simulink library "simetranss"  (R2024b)
settings: Solver=VariableStepAuto  StartTime=0.0  StopTime=10.0  RelTol=1e-3
PostLoadFcn:
  | Ts=1e-6
InitFcn:
  | Ts=1e-6
undefined symbols (not defined in the file): C, C_601, C_603, C_606, CC, Csnu, Csnubber, DiscIntNeverNeededParam, DPL, DPL1ph, FluxTable, ft2km, gcbh, h, Half, Imap2, L, L_601, L_603, L_606, Lbase, LpejoSw, Newton, R_601, R_603, R_606, Raphson, ResistanceM, Roff, Ron, RotorAngles, Rsnu, Rsnubber, Rt4, SampleTime, simetran, sps, sps_rtmsupport, StatorCurrents, T_2wind_ratio, T_Lpu, T_Lpu_pri, T_Rpu, T_Rpu_pri, T_Vpri, T_Vpri_15comp, T_Vsec, Ti, Ts_Power, Z, Zbase, Zm
libraries: fl_lib x248, ee_lib x146, nesl_utility x122, $bdroot x29, simulink x15, eeGeneralControl x2, spsStairGeneratorLib x2, artemis x1
(part 6 of 12)

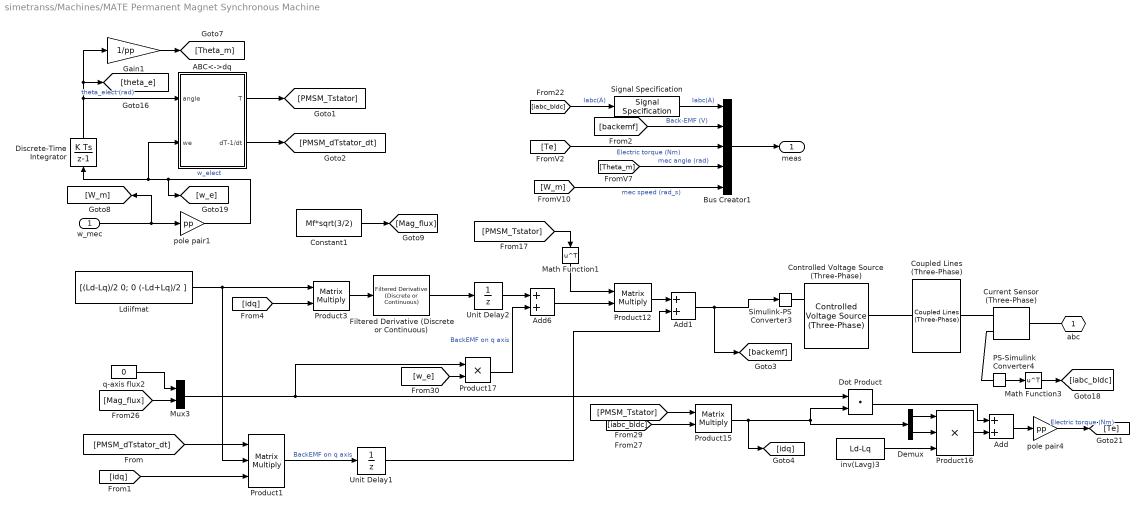
== system simetranss/Machines/MATE Permanent Magnet Synchronous Machine ==
  "   w_mec" : Inport
  ABC<->dq : Subsystem
  Add : Sum
  Add1 : Sum  Inputs=2
  Add6 : Sum  Inputs=2
  Bus Creator1 : BusCreator  Inputs=5
  Constant1 : Constant  Value=Mf*sqrt(3/2)
  Controlled Voltage Source (Three-Phase) : ee_lib/Sources/Controlled Voltage Source (Three-Phase)  input_option=ee.enum.inputType.instantaneous  FRated=60 Hz
      settings: InternalSimscapePortConfiguration="{\"Bottom\":[],\"Left\":[{\"id\":\"S\",\"label\":\"S\",\"type\":\"input\"},{\"id\":\"n\",\"label\":\"n\",\"type\":\"foundation.electrical.electrical\"}],\"Right\":[{\"id\":\"N\",\"label\":\"~\",\"type\":\"foundation.electrical.three_phase\"}],\"Top\":[]}"
  Coupled Lines (Three-Phase) : ee_lib/Passive/Lines/Coupled Lines (Three-Phase)  prm=1  La=1e-3 H  Lb=1e-3 H  Lc=1e-3 H  L=Ld+Lq H  Lmab=3e-4 H  Lmac=3e-4 H  Lmbc=3e-4 H  Lm=(Ld+Lq)/2 H  Ra=0.001 Ohm  Rb=0.001 Ohm  Rc=0.001 Ohm  R=Rs Ohm  Rm=0 Ohm  Ga=1e-9 1/Ohm  Gb=1e-9 1/Ohm  Gc=1e-9 1/Ohm  G=1e-9 1/Ohm  I_L_specify=off  I_L_priority=High  I_L=[0, 0, 0] A  I_L_nominal_specify=off  I_L_nominal_value=1  I_L_nominal_unit=A  i_La_specify=off  i_La_priority=High  i_La=0 A  i_La_nominal_specify=off  i_La_nominal_value=1  i_La_nominal_unit=A  i_Lb_specify=off  i_Lb_priority=High  i_Lb=0 A  i_Lb_nominal_specify=off  i_Lb_nominal_value=1  i_Lb_nominal_unit=A  i_Lc_specify=off  i_Lc_priority=High  i_Lc=0 A  i_Lc_nominal_specify=off  i_Lc_nominal_value=1  i_Lc_nominal_unit=A
      settings: InternalSimscapePortConfiguration="{\"Bottom\":[],\"Left\":[{\"id\":\"N1\",\"label\":\"~1\",\"type\":\"foundation.electrical.three_phase\"}],\"Right\":[{\"id\":\"N2\",\"label\":\"~2\",\"type\":\"foundation.electrical.three_phase\"}],\"Top\":[]}"
  Current Sensor (Three-Phase) : ee_lib/Sensors & Transducers/Current Sensor (Three-Phase)
  Demux : Demux  Outputs=2
  Discrete-Time Integrator : DiscreteIntegrator  InitialCondition=pp*AngInit/180*pi  SampleTime=Ts  ICPrevOutput=DiscIntNeverNeededParam  ICPrevScaledInput=DiscIntNeverNeededParam
  Dot Product : DotProduct  OutDataTypeStr=Inherit: Inherit via internal rule
  Filtered Derivative (Discrete or Continuous) : eeGeneralControl/Filtered Derivative (Discrete or Continuous)  K=1  T=sal_der  B=inf  A=-inf  minRatio=10  init_option=Inherited from block input  x0=0  Ts=Ts
  Gain1 : Gain  Gain=1/pp
  Ldiifmat : Constant  Value=[(Ld-Lq)/2 0; 0 (-Ld+Lq)/2 ]
  Math Function1 : Math  Operator=transpose  SignedPower=on
  Math Function3 : Math  Operator=transpose  SignedPower=on
  Mux3 : Mux  Inputs=2
  PS-Simulink Converter4 : nesl_utility/PS-Simulink Converter  PhysicalDomain=network_engine_domain  SubClassName=ps_output  LeftPortType=input  RightPortType=output  PseudoPeriodic=off  Frequencies=[]  VectorFormat=inherit  Unit=inherit  AffineConversion=off
  Product1 : Product  Inputs=3  Multiplication=Matrix(*)  SaturateOnIntegerOverflow=on  OutDataTypeStr=Inherit: Same as first input
  Product12 : Product  Multiplication=Matrix(*)  SaturateOnIntegerOverflow=on  OutDataTypeStr=Inherit: Same as first input
  Product15 : Product  Multiplication=Matrix(*)  SaturateOnIntegerOverflow=on  OutDataTypeStr=Inherit: Same as first input
  Product16 : Product  Inputs=3  SaturateOnIntegerOverflow=on  OutDataTypeStr=Inherit: Same as first input
  Product17 : Product  RndMeth=Zero
  Product3 : Product  Multiplication=Matrix(*)  SaturateOnIntegerOverflow=on  OutDataTypeStr=Inherit: Same as first input
  Signal Specification : SignalSpecification  Dimensions=3
  Simulink-PS Converter3 : nesl_utility/Simulink-PS Converter  PhysicalDomain=network_engine_domain  SubClassName=ps_input  LeftPortType=input  RightPortType=output  PseudoPeriodic=off  Frequencies=[]  NoiseDistribution=none  NoiseParameters=[]  Unit=1  AffineConversion=off  FilteringAndDerivatives=provide  SimscapeFilterOrder=1  InputFilterTimeConstant=0.001  UdotUserProvided=0
  Unit Delay1 : UnitDelay  SampleTime=Ts  HasFrameUpgradeWarning=on
  Unit Delay2 : UnitDelay  SampleTime=Ts  HasFrameUpgradeWarning=on
  inv(Lavg)3 : Constant  Value=Ld-Lq
  pole pair1 : Gain  Gain=pp
  pole pair4 : Gain  Gain=pp
  q-axis flux2 : Constant  Value=0
  "   abc" : PMIOPort  Side=Left
  meas : Outport  VectorParamsAs1DForOutWhenUnconnected=off
  wires:
  Unit Delay1/1 -> Add1/2
  [idq] -> Product3/2
  Product1/1 -> Unit Delay1/1  "BackEMF on q axis"
  Add1/1 -> Simulink-PS Converter3/1, [backemf]
  Product12/1 -> Add1/1
  [idq] -> Product1/3
  Ldiifmat/1 -> Product3/1, Product1/2
  [PMSM_dTstator_dt] -> Product1/1
  Add6/1 -> Product12/2
  Math Function1/1 -> Product12/1
  [PMSM_Tstator] -> Product15/1
  [iabc_bldc] -> Product15/2
  Math Function3/1 -> [iabc_bldc]
  [PMSM_Tstator] -> Math Function1/1
  ABC<->dq/2(dT-1/dt) -> [PMSM_dTstator_dt]
  Product17/1 -> Add6/2  "BackEMF on q axis"
  Unit Delay2/1 -> Add6/1
  Mux3/1 -> Product17/1, Dot Product/1
  [w_e] -> Product17/2
  Dot Product/1 -> Add/1
  Add/1 -> pole pair4/1
  Product16/1 -> Add/2
  pole pair4/1 -> [Te]  "Electric torque (Nm)"
  Demux/2 -> Product16/2
  Demux/1 -> Product16/1
  inv(Lavg)3/1 -> Product16/3
  Product15/1 -> Demux/1, Dot Product/2, [idq]
  Filtered Derivative (Discrete or Continuous)/1 -> Unit Delay2/1
  q-axis flux2/1 -> Mux3/1
  [Mag_flux] -> Mux3/2
  Product3/1 -> Filtered Derivative (Discrete or Continuous)/1
  [Te] -> Bus Creator1/3  "Electric torque (Nm)"
  [Theta_m] -> Bus Creator1/4  "mec angle (rad)"
  PS-Simulink Converter4/1 -> Math Function3/1
  [backemf] -> Bus Creator1/2  "Back-EMF (V)"
  Bus Creator1/1 -> meas/1
  Signal Specification/1 -> Bus Creator1/1  "Iabc(A)"
  [W_m] -> Bus Creator1/5  "mec speed (rad_s)"
  [iabc_bldc] -> Signal Specification/1  "Iabc(A)"
  Gain1/1 -> [Theta_m]
  Discrete-Time Integrator/1 -> ABC<->dq/1(angle), [theta_e], Gain1/1  "theta_elect (rad)"
  pole pair1/1 -> Discrete-Time Integrator/1, ABC<->dq/2(we), [w_e]  "w_elect"
  "   w_mec"/1 -> [W_m], pole pair1/1
  ABC<->dq/1(T) -> [PMSM_Tstator]
  Constant1/1 -> [Mag_flux]
  connections:
  PS-Simulink Converter4/LConn1 -- Current Sensor (Three-Phase)/RConn1
  Controlled Voltage Source (Three-Phase)/RConn1 -- Coupled Lines (Three-Phase)/RConn1
  Coupled Lines (Three-Phase)/LConn1 -- Current Sensor (Three-Phase)/RConn2
  Simulink-PS Converter3/RConn1 -- Controlled Voltage Source (Three-Phase)/LConn1
  Current Sensor (Three-Phase)/LConn1 -- "   abc"/RConn1

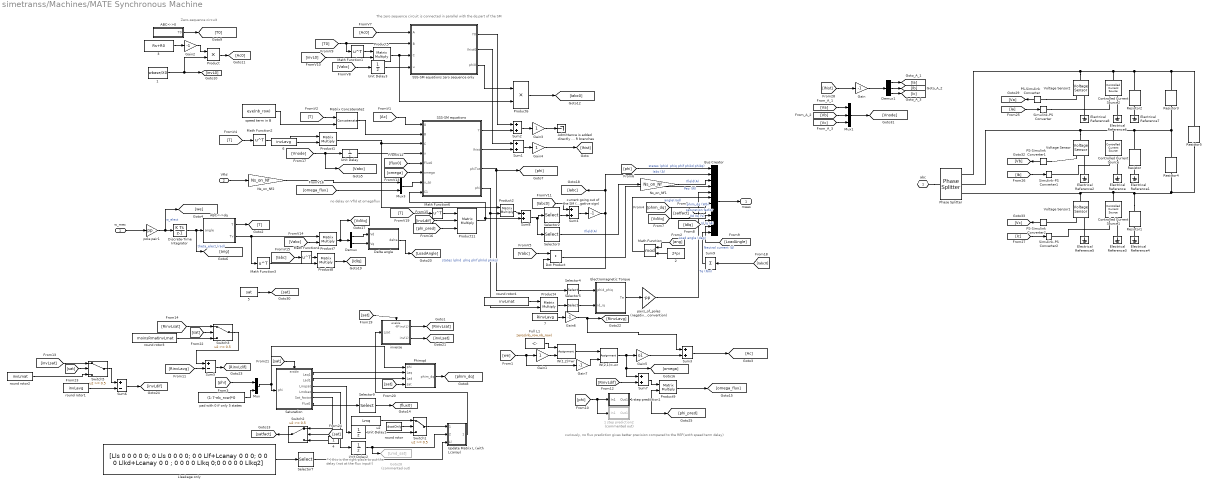
== system simetranss/Machines/MATE Synchronous Machine ==
  note: no delay on Vfld et omegaflux
  note: curiously, no flux prediction gives better precision compared to the REF(woth speed term delay)
  note: The zero sequence circuit is connected in parallel with the dq part of the SM
  note: Zero-sequence circuit
  note: ^
      | |
      | this is the right place to put the delay
      | (not at the flux input!)
  "   w_mec" : Inport
  "   Vfld" : Inport  Port=2
  1 : Constant  Value=wbase/X0
  1 step prediction1 : Subsystem
  1 step prediction2 : Subsystem  Commented=on
  2 : Constant  Value=2*pi
  3 : Constant  Value=Rs+R0
  4 : Constant
  5 : Constant  Value=sat
  6 : Constant  Value=invLavg
  7 : Constant  Value=RinvLavg
  ABC<->0 : Subsystem
  ABC<->dq : Subsystem
  Admittance is added directly with R branches : Terminator
  Bus Creator : BusCreator  Inputs=12
  Controlled Current Source : fl_lib/Electrical/Electrical Sources/Controlled Current Source
  Controlled Current Source1 : fl_lib/Electrical/Electrical Sources/Controlled Current Source
  Controlled Current Source2 : fl_lib/Electrical/Electrical Sources/Controlled Current Source
  Delta angle : Subsystem
  Demux : Demux  Outputs=2
  Demux1 : Demux  Outputs=3
      settings: DisplayOption=none
  Discrete-Time Integrator : DiscreteIntegrator  InitialCondition=theta_0  SampleTime=Ts  ICPrevOutput=DiscIntNeverNeededParam  ICPrevScaledInput=DiscIntNeverNeededParam
  Dot Product : DotProduct  OutDataTypeStr=Inherit: Inherit via internal rule
  Electrical Reference{,1..8} (9 alike) : fl_lib/Electrical/Electrical Elements/Electrical Reference
  Electromagnetic Torque : Subsystem
  Full L1 : Constant  Value=zeros(nb_row,nb_row)
  Gain : Gain  Gain=-1
  Gain1 : Gain  SaturateOnIntegerOverflow=on  OutDataTypeStr=Inherit: Same as input  ParamDataTypeStr=Inherit: Same as input
  Gain2 : Gain  Gain=-1
  Gain3 : Gain
  Gain4 : Gain
  Gain5 : Gain  Gain=o1
  Gain6 : Gain  Gain=-1
  Gain7 : Gain  Gain=-1  SaturateOnIntegerOverflow=on  OutDataTypeStr=Inherit: Same as input  ParamDataTypeStr=Inherit: Same as input
  Goto28 : Goto  Commented=on  GotoTag=Lmd_sat
  Lleakage only : Constant  Value="[Lls 0 0 0 0 0; 0 Lls 0 0  0 0; 0 0 Llf+Lcanay 0 0 0; 0 0 0 Llkd+Lcanay 0 0 ; 0 0 0 0 Llkq 0;0 0 0 0 0 Llkq2]"
  Math Function : Math  Operator=mod  SignedPower=on
  Math Function{1..4,6} (5 alike) : Math  Operator=transpose  SignedPower=on
  Matrix Concatenate2 : Concatenate  Mode=Multidimensional array  ConcatenateDimension=2
  Mux : Mux  Inputs=2
  Mux1 : Mux  Inputs=3
  Mux3 : Mux  Inputs=2
  Ns_on_Nf1 : Gain  Gain=Ns_on_Nf
  Ns_on_Nf2 : Gain  Gain=Ns_on_Nf
  PS-Simulink Converter : nesl_utility/PS-Simulink Converter  PhysicalDomain=network_engine_domain  SubClassName=ps_output  LeftPortType=input  RightPortType=output  PseudoPeriodic=off  Frequencies=[]  VectorFormat=inherit  Unit=inherit  AffineConversion=off
  PS-Simulink Converter1 : nesl_utility/PS-Simulink Converter  PhysicalDomain=network_engine_domain  SubClassName=ps_output  LeftPortType=input  RightPortType=output  PseudoPeriodic=off  Frequencies=[]  VectorFormat=inherit  Unit=inherit  AffineConversion=off
  PS-Simulink Converter2 : nesl_utility/PS-Simulink Converter  PhysicalDomain=network_engine_domain  SubClassName=ps_output  LeftPortType=input  RightPortType=output  PseudoPeriodic=off  Frequencies=[]  VectorFormat=inherit  Unit=inherit  AffineConversion=off
  Phase Splitter : ee_lib/Connectors & References/Phase Splitter
  Phimqd : Subsystem
  Product : Product  RndMeth=Zero
  Product{1..2,4..5,7..9} (7 alike) : Product  Multiplication=Matrix(*)  SaturateOnIntegerOverflow=on  OutDataTypeStr=Inherit: Same as first input
  Product11 : Product  Inputs=3  Multiplication=Matrix(*)  SaturateOnIntegerOverflow=on  OutDataTypeStr=Inherit: Same as first input
  Product6 : Product  SaturateOnIntegerOverflow=on  OutDataTypeStr=Inherit: Same as first input
  Resistor : fl_lib/Electrical/Electrical Elements/Resistor  R=ResistanceM(2,2) Ohm  i_specify=off  i_priority=None  i=0 A  i_nominal_specify=off  i_nominal_value=1  i_nominal_unit=A  v_specify=off  v_priority=None  v=0 V  v_nominal_specify=off  v_nominal_value=1  v_nominal_unit=V
  Resistor1 : fl_lib/Electrical/Electrical Elements/Resistor  R=ResistanceM(3,3) Ohm  i_specify=off  i_priority=None  i=0 A  i_nominal_specify=off  i_nominal_value=1  i_nominal_unit=A  v_specify=off  v_priority=None  v=0 V  v_nominal_specify=off  v_nominal_value=1  v_nominal_unit=V
  Resistor2 : fl_lib/Electrical/Electrical Elements/Resistor  R=ResistanceM(1,1) Ohm  i_specify=off  i_priority=None  i=0 A  i_nominal_specify=off  i_nominal_value=1  i_nominal_unit=A  v_specify=off  v_priority=None  v=0 V  v_nominal_specify=off  v_nominal_value=1  v_nominal_unit=V
  Resistor3 : fl_lib/Electrical/Electrical Elements/Resistor  R=ResistanceM(1,2) Ohm  i_specify=off  i_priority=None  i=0 A  i_nominal_specify=off  i_nominal_value=1  i_nominal_unit=A  v_specify=off  v_priority=None  v=0 V  v_nominal_specify=off  v_nominal_value=1  v_nominal_unit=V
  Resistor4 : fl_lib/Electrical/Electrical Elements/Resistor  R=ResistanceM(2,3) Ohm  i_specify=off  i_priority=None  i=0 A  i_nominal_specify=off  i_nominal_value=1  i_nominal_unit=A  v_specify=off  v_priority=None  v=0 V  v_nominal_specify=off  v_nominal_value=1  v_nominal_unit=V
  Resistor5 : fl_lib/Electrical/Electrical Elements/Resistor  R=ResistanceM(1,3) Ohm  i_specify=off  i_priority=None  i=0 A  i_nominal_specify=off  i_nominal_value=1  i_nominal_unit=A  v_specify=off  v_priority=None  v=0 V  v_nominal_specify=off  v_nominal_value=1  v_nominal_unit=V
  SSS-SM equations : Subsystem
  SSS-SM equations zero sequence only : Subsystem
  Saturation : Subsystem
  Selector2 : Selector  InputPortWidth=4  IndexOptions=Index vector (dialog)  Indices=[1 2 3 ]  OutputSizes=1
  Selector3 : Selector  InputPortWidth=4  IndexOptions=Index vector (dialog)  Indices=[4 ]  OutputSizes=1
  Selector4 : Selector  InputPortWidth=nb_row  IndexOptions=Index vector (dialog)  Indices=[1 2]  OutputSizes=1
  Selector5 : Selector  InputPortWidth=nb_row  IndexOptions=Index vector (dialog)  Indices=[1 2]  OutputSizes=1
  Selector7 : Selector  NumberOfDimensions=2  InputPortWidth=3  IndexOptions=Index vector (dialog),Index vector (dialog)  Indices=[1:nb_row],[1:nb_row]  OutputSizes=1,1
  Selector9 : Selector  InputPortWidth=6  IndexOptions=Index vector (dialog)  Indices=[1:nb_row]  OutputSizes=1
  Simulink-PS Converter : nesl_utility/Simulink-PS Converter  PhysicalDomain=network_engine_domain  SubClassName=ps_input  LeftPortType=input  RightPortType=output  PseudoPeriodic=off  Frequencies=[]  NoiseDistribution=none  NoiseParameters=[]  Unit=1  AffineConversion=off  FilteringAndDerivatives=provide  SimscapeFilterOrder=1  InputFilterTimeConstant=0.001  UdotUserProvided=0
  Simulink-PS Converter1 : nesl_utility/Simulink-PS Converter  PhysicalDomain=network_engine_domain  SubClassName=ps_input  LeftPortType=input  RightPortType=output  PseudoPeriodic=off  Frequencies=[]  NoiseDistribution=none  NoiseParameters=[]  Unit=1  AffineConversion=off  FilteringAndDerivatives=provide  SimscapeFilterOrder=1  InputFilterTimeConstant=0.001  UdotUserProvided=0
  Simulink-PS Converter2 : nesl_utility/Simulink-PS Converter  PhysicalDomain=network_engine_domain  SubClassName=ps_input  LeftPortType=input  RightPortType=output  PseudoPeriodic=off  Frequencies=[]  NoiseDistribution=none  NoiseParameters=[]  Unit=1  AffineConversion=off  FilteringAndDerivatives=provide  SimscapeFilterOrder=1  InputFilterTimeConstant=0.001  UdotUserProvided=0
  Sum{1..4,7..8} (6 alike) : Sum  SaturateOnIntegerOverflow=on
  Sum5 : Sum  Inputs=+-  SaturateOnIntegerOverflow=on
  Sum6 : Sum  Inputs=+-  SaturateOnIntegerOverflow=on
  Sum9 : Sum  Inputs=+  SaturateOnIntegerOverflow=on
  Switch{1..3,5} (4 alike) : Switch  Threshold=0.5  SaturateOnIntegerOverflow=off  InputSameDT=off
  Unit Delay : UnitDelay  SampleTime=Ts  HasFrameUpgradeWarning=on
  Unit Delay1 : UnitDelay  InitialCondition=Lmq  SampleTime=Ts  HasFrameUpgradeWarning=on
  Unit Delay2 : UnitDelay  InitialCondition=Lmd  SampleTime=Ts  HasFrameUpgradeWarning=on
  Unit Delay3 : UnitDelay  SampleTime=Ts  HasFrameUpgradeWarning=on
  Update Matrix L (with Lcanay) : Subsystem
  Voltage Sensor : fl_lib/Electrical/Electrical Sensors/Voltage Sensor
  Voltage Sensor1 : fl_lib/Electrical/Electrical Sensors/Voltage Sensor
  Voltage Sensor2 : fl_lib/Electrical/Electrical Sensors/Voltage Sensor
  W(1,2)=wr : Assignment  NumberOfDimensions=2  IndexOptions=Index vector (dialog),Index vector (dialog)  Indices=1,2  OutputSizes=1,1
  W(2,1)=-wr : Assignment  NumberOfDimensions=2  IndexOptions=Index vector (dialog),Index vector (dialog)  Indices=2,1  OutputSizes=1,1
  current going out of the SM (negative sign) : Gain  Gain=-1
  inverse : Subsystem
  pad with 0 if only 5 states : Constant  Value=(1:7-nb_row)*0
  pairs_of_poles (negative sign for generator convention) : Gain  Gain=-pp
  pole pair1 : Gain  Gain=pp
  round rotor : Constant  Value=dsatOnly
  round rotor1 : Constant  Value=invLavg
  round rotor2 : Constant  Value=invLmat
  round rotor3 : Constant  Value=moinsRmatinvLmat
  round rotor4 : Constant  Value=invLmat
  speed term in B : Constant  Value=eye(nb_row)  VectorParams1D=off
  u2 : Constant  Value=Lmq
  "abc   " : PMIOPort  Side=Right
  "meas   " : Outport
  wires:
  Product6/1 -> [Iabc0]
  SSS-SM equations zero sequence only/3(phi0) -> Product6/1
  Gain4/1 -> [Ihist]
  [Ia] -> Simulink-PS Converter/1
  [Ib] -> Simulink-PS Converter1/1
  PS-Simulink Converter2/1 -> [Vc]
  [Vb] -> Mux1/2
  [Ihist] -> Gain/1
  [Va] -> Mux1/1
  Demux1/3 -> [Ic]
  [Ic] -> Simulink-PS Converter2/1
  PS-Simulink Converter/1 -> [Va]
  Gain/1 -> Demux1/1
  [Vc] -> Mux1/3
  Demux1/1 -> [Ia]
  Demux1/2 -> [Ib]
  Mux1/1 -> [Vnode]
  PS-Simulink Converter1/1 -> [Vb]
  SSS-SM equations/4(phi) -> Product4/2, Product2/2
  Selector9/1 -> [flux0]
  [phi] -> Bus Creator/1  "states (phid  phiq phif phikd phikq)"
  [omega] -> SSS-SM equations/6(omega)
  Full L1/1 -> W(1,2)=wr/1
  Sum3/1 -> [Ac]
  W(2,1)=-wr/1 -> Gain5/1, Sum7/1, [omega]
  [flux0] -> SSS-SM equations/5(Flux0)
  Saturation/6(Flux0) -> Selector9/1
  4/1 -> Switch2/3
  Saturation/5(Sat_factor) -> Switch2/1
  Switch2/1 -> [satfact]
  [satfact] -> Bus Creator/8  "saturation factor"
  Sum4/1 -> current going out of the SM (negative sign)/1
  Selector2/1 -> Sum4/2
  Sum2/1 -> Gain3/1
  SSS-SM equations/1(Y) -> Sum2/2
  SSS-SM equations/2(Ihist) -> Sum1/2
  Sum1/1 -> Gain4/1
  Product5/1 -> SSS-SM equations zero sequence only/3(C), Product6/2
  [invL0] -> Product5/2
  Math Function1/1 -> Product5/1
  [T0] -> SSS-SM equations zero sequence only/2(B), Math Function1/1
  Unit Delay3/1 -> SSS-SM equations zero sequence only/4(u)
  [Vabc] -> Unit Delay3/1
  [Ac0] -> SSS-SM equations zero sequence only/1(A)
  Product/1 -> [Ac0]
  1/1 -> Product/2, [invL0]
  Gain2/1 -> Product/1
  3/1 -> Gain2/1
  ABC<->0/1(T0) -> [T0]
  Mux/1 -> Phimqd/1(phi), Saturation/1(phi)
  pad with 0 if only 5 states/1 -> Mux/2
  [Ac] -> SSS-SM equations/1(A)
  Selector7/1 -> Update Matrix L (with Lcanay)/3(Ll)
  u2/1 -> Switch1/1
  Unit Delay1/1 -> Switch1/3
  Phimqd/1(phim_dq) -> [phim_dq]
  [phim_dq] -> Bus Creator/7  "phim_dq (Wb)"
  Lleakage only/1 -> Selector7/1
  Unit Delay2/1 -> Update Matrix L (with Lcanay)/2(Lmd), Goto28/1
  round rotor/1 -> Switch1/2
  Switch1/1 -> Update Matrix L (with Lcanay)/1(Lmq)
  Saturation/4(Lmdsat) -> Unit Delay2/1
  Saturation/3(Lmqsat) -> Unit Delay1/1
  Saturation/2(Lad1) -> Phimqd/3(Lad)
  Saturation/1(Laq1) -> Phimqd/2(Laq)
  [phi] -> Mux/1
  2/1 -> Math Function/2
  Math Function/1 -> Bus Creator/6  "angle(rad)"
  [ang] -> Math Function/1
  "   w_mec"/1 -> pole pair1/1
  current going out of the SM (negative sign)/1 -> Dot Product/2, Bus Creator/2, [Iabc]  "Iabc (A)"
  Dot Product/1 -> Bus Creator/4  "Peo (W)"
  [Vabc] -> Dot Product/1
  pairs_of_poles (negative sign for generator convention)/1 -> Bus Creator/5  "Te (Nm)"
  Product4/1 -> Selector5/1
  Selector4/1 -> Electromagnetic Torque/1(phid_phiq)
  Selector5/1 -> Electromagnetic Torque/2(id_iq)
  Electromagnetic Torque/1(Te) -> pairs_of_poles (negative sign for generator convention)/1
  Selector3/1 -> Ns_on_Nf1/1  "Ifield(A)"
  Gain1/1 -> W(1,2)=wr/2
  Math Function2/1 -> Product1/1
  Product1/1 -> SSS-SM equations/3(C), Product2/1
  [T] -> Math Function2/1
  [we] -> Gain7/1, Gain1/1
  W(1,2)=wr/1 -> W(2,1)=-wr/1
  Gain7/1 -> W(2,1)=-wr/2
  Unit Delay/1 -> SSS-SM equations/4(u)
  SSS-SM equations/3(phiTot) -> Selector4/1, [phi]  "states (phid  phiq phif phikd phikq)"
  Discrete-Time Integrator/1 -> [ang], ABC<->dq/1(angle)  "theta_elect (rad)"
  ABC<->dq/1(T) -> [T]
  pole pair1/1 -> Discrete-Time Integrator/1, [we]  "w_elect"
  Product7/1 -> [VdVq], Demux/1
  Demux/2 -> Delta angle/2(Vq)
  Demux/1 -> Delta angle/1(Vd)
  [Vabc] -> Product7/2
  Delta angle/1(delta) -> [LoadAngle]
  Product8/1 -> [IdIq]
  [Iabc] -> Math Function4/1
  Math Function3/1 -> Product8/2
  Math Function4/1 -> Product8/1
  [VdVq] -> Bus Creator/9  "Vd Vq (V)"
  [IdIq] -> Bus Creator/10  "Id Iq (A)"
  [LoadAngle] -> Bus Creator/11  "Load angle (deg)"
  ABC<->dq/2(Tv) -> Math Function3/1, Product7/1
  Gain5/1 -> Sum3/2
  [T] -> Matrix Concatenate2/1
  speed term in B/1 -> Matrix Concatenate2/2
  Matrix Concatenate2/1 -> SSS-SM equations/2(B)
  Bus Creator/1 -> "meas   "/1
  Product9/1 -> [omega_flux]
  Ns_on_Nf1/1 -> Bus Creator/3  "Ifield(A)"
  7/1 -> Gain6/1
  [RinvLavg] -> Sum5/2
  Gain6/1 -> Sum3/1, [RinvLavg]
  Sum5/1 -> [RinvLdif]
  [RinvLdif] -> Sum7/2
  Sum7/1 -> Product9/1
  6/1 -> Product1/2
  round rotor1/1 -> Sum6/2
  Sum6/1 -> [invLdif]
  [T] -> Math Function6/1
  Math Function6/1 -> Product11/1
  [invLdif] -> Product11/2
  [phi_pred] -> Product11/3
  [Iabc0] -> Sum4/1
  Product2/1 -> Sum8/1
  Sum8/1 -> Selector3/1, Selector2/1
  Product11/1 -> SSS-SM equations/8(C1), Sum8/2
  round rotor4/1 -> Product4/1
  [omega_flux] -> Mux3/2
  [phi] -> 1 step prediction1/1(In1), 1 step prediction2/1(In1)
  SSS-SM equations zero sequence only/1(Y0) -> Sum2/1
  SSS-SM equations zero sequence only/2(Ihist0) -> Sum1/1
  [Vnode] -> [Vabc], Unit Delay/1
  [Iabc0] -> Sum9/1
  Sum9/1 -> Bus Creator/12  "Neutral current (A)"
  Update Matrix L (with Lcanay)/1(Lsat) -> inverse/1(Lsat)
  inverse/1(-R*inv(L)) -> [RinvLsat]
  round rotor3/1 -> Switch3/3
  [RinvLsat] -> Switch3/1
  Switch3/1 -> Sum5/1
  Ns_on_Nf2/1 -> Mux3/1
  "   Vfld"/1 -> Ns_on_Nf2/1
  Gain3/1 -> Admittance is added directly with R branches/1
  inverse/2(inv(L)) -> [invLsat]
  round rotor2/1 -> Switch5/3
  [invLsat] -> Switch5/1
  5/1 -> [sat]
  [sat] -> inverse/Enable
  [sat] -> Phimqd/4(sat)
  [sat] -> Saturation/Enable
  [sat] -> Switch3/2
  [sat] -> Switch5/2
  Switch5/1 -> Sum6/1
  [sat] -> Switch2/2
  1 step prediction1/1(Out1) -> [phi_pred], Product9/2
  Mux3/1 -> SSS-SM equations/7(u_sp)
  connections:
  Electrical Reference5/LConn1 -- Voltage Sensor1/RConn2
  Electrical Reference8/LConn1 -- Voltage Sensor2/RConn2
  PS-Simulink Converter/LConn1 -- Voltage Sensor2/RConn1
  Controlled Current Source/RConn1 -- Simulink-PS Converter1/RConn1
  Voltage Sensor1/RConn1 -- PS-Simulink Converter2/LConn1
  Electrical Reference/LConn1 -- Controlled Current Source/RConn2
  Simulink-PS Converter/RConn1 -- Controlled Current Source2/RConn1
  PS-Simulink Converter1/LConn1 -- Voltage Sensor/RConn1
  Electrical Reference6/LConn1 -- Controlled Current Source2/RConn2
  Electrical Reference4/LConn1 -- Resistor1/RConn1
  "abc   "/RConn1 -- Phase Splitter/LConn1
  Controlled Current Source1/RConn1 -- Simulink-PS Converter2/RConn1
  Electrical Reference7/LConn1 -- Resistor2/RConn1
  Electrical Reference1/LConn1 -- Resistor/RConn1
  Electrical Reference3/LConn1 -- Controlled Current Source1/RConn2
  Electrical Reference2/LConn1 -- Voltage Sensor/RConn2
  Voltage Sensor2/LConn1 -- Phase Splitter/RConn1 -- Controlled Current Source2/LConn1 -- Resistor2/LConn1 -- Resistor5/LConn1 -- Resistor3/LConn1
  Resistor1/LConn1 -- Voltage Sensor1/LConn1 -- Phase Splitter/RConn3 -- Controlled Current Source1/LConn1 -- Resistor5/RConn1 -- Resistor4/RConn1
  Voltage Sensor/LConn1 -- Phase Splitter/RConn2 -- Resistor/LConn1 -- Resistor3/RConn1 -- Resistor4/LConn1 -- Controlled Current Source/LConn1

== system simetranss/Machines/Mechanical model ==
  note: Pm=Tm*w so a divider by w can be added if Pm is provided instead of Tm
  Te : Inport  PortDimensions=1
  Tm : Inport  Port=2
  1 ----- J : Gain  Gain=1/J  SaturateOnIntegerOverflow=on  OutDataTypeStr=Inherit: Same as input  ParamDataTypeStr=Inherit: Same as input
  F : Gain  Gain=F  SaturateOnIntegerOverflow=on  OutDataTypeStr=Inherit: Same as input  ParamDataTypeStr=Inherit: Same as input
  Rotor speed interator : DiscreteIntegrator  InitialCondition=fo*2*pi  SampleTime=Ts  ICPrevOutput=DiscIntNeverNeededParam  ICPrevScaledInput=DiscIntNeverNeededParam
  Sum2 : Sum  Inputs=-+-  InputSameDT=on  SaturateOnIntegerOverflow=on  OutDataTypeStr=Inherit: Same as first input
  wmec : Outport  InitialOutput=0  VectorParamsAs1DForOutWhenUnconnected=off
  wires:
  Tm/1 -> Sum2/1  "Tm"
  Sum2/1 -> 1 ----- J/1
  F/1 -> Sum2/3
  Te/1 -> Sum2/2  "Te"
  1 ----- J/1 -> Rotor speed interator/1
  Rotor speed interator/1 -> wmec/1, F/1  "w"

== system simetranss/Measure/Bus Measure ==
  Measure : Subsystem
  Pass : Subsystem  Commented=on
  + : PMIOPort  Side=Left
  - : PMIOPort  Port=2  Side=Right
  connections:
  +/RConn1 -- Measure/LConn1 -- Pass/LConn1
  -/RConn1 -- Measure/RConn1 -- Pass/RConn1

== system simetranss/Measure/Current Mesure ==
  Current Sensor : fl_lib/Electrical/Electrical Sensors/Current Sensor
  PS-Simulink Converter : nesl_utility/PS-Simulink Converter  PhysicalDomain=network_engine_domain  SubClassName=ps_output  LeftPortType=input  RightPortType=output  PseudoPeriodic=off  Frequencies=[]  VectorFormat=inherit  Unit=inherit  AffineConversion=off
  + : PMIOPort  Side=Left
  - : PMIOPort  Port=2  Side=Right
  tag scope: Ia=global
  wires:
  PS-Simulink Converter/1 -> [Ia]
  connections:
  Current Sensor/RConn2 -- -/RConn1
  Current Sensor/LConn1 -- +/RConn1
  Current Sensor/RConn1 -- PS-Simulink Converter/LConn1

== system simetranss/Measure/Voltage Mesure ==
  PS-Simulink Converter : nesl_utility/PS-Simulink Converter  PhysicalDomain=network_engine_domain  SubClassName=ps_output  LeftPortType=input  RightPortType=output  PseudoPeriodic=off  Frequencies=[]  VectorFormat=inherit  Unit=inherit  AffineConversion=off
  Voltage Sensor : fl_lib/Electrical/Electrical Sensors/Voltage Sensor
  + : PMIOPort  Side=Left
  - : PMIOPort  Port=2  Side=Right
  tag scope: Va=global
  wires:
  PS-Simulink Converter/1 -> [Va]
  connections:
  Voltage Sensor/RConn1 -- PS-Simulink Converter/LConn1
  +/RConn1 -- Voltage Sensor/LConn1
  Voltage Sensor/RConn2 -- -/RConn1

== system simetranss/Measure/bus ==
  Connection Port : PMIOPort  Side=Left
  Connection Port1 : PMIOPort  Port=2  Side=Right
  connections:
  Connection Port/RConn1 -- Connection Port1/RConn1

== system simetranss/Measure/bus2 ==
  Connection Port : PMIOPort  Side=Left
  Connection Port1 : PMIOPort  Port=2  Side=Right
  Connection Port2 : PMIOPort  Port=3  Side=Left
  Connection Port3 : PMIOPort  Port=4  Side=Right
  connections:
  Connection Port2/RConn1 -- Connection Port3/RConn1
  Connection Port/RConn1 -- Connection Port1/RConn1

== system simetranss/Misc/Discrete Mean value ==
  In : Inport  SampleTime=Ts
  Model : Subsystem
  Mean : Outport  SampleTime=Ts  VectorParamsAs1DForOutWhenUnconnected=off
  wires:
  Model/1(Mean) -> Mean/1
  In/1 -> Model/1(In)

== system simetranss/Misc/Fourier ==
  In : Inport  SampleTime=Ts
  Complex to Magnitude-Angle : ComplexToMagnitudeAngle
  Discrete Mean value : $bdroot/Misc/Discrete Mean value  Freq=mate.Freq  Vinit=mate.Real_Init  Ts=Ts
  Discrete Mean value1 : $bdroot/Misc/Discrete Mean value  Freq=mate.Freq  Vinit=mate.Imag_Init  Ts=Ts
  Product : Product  InputSameDT=on  SaturateOnIntegerOverflow=on  OutDataTypeStr=Inherit: Same as first input
  Product1 : Product  InputSameDT=on  SaturateOnIntegerOverflow=on  OutDataTypeStr=Inherit: Same as first input
  Rad->Deg. : Gain  Gain=180/pi  SaturateOnIntegerOverflow=on  OutDataTypeStr=Inherit: Same as input  ParamDataTypeStr=Inherit: Same as input
  Real-Imag to Complex : RealImagToComplex
  cos(wt) : Sin  Amplitude=sps.k  Frequency=2*pi*Freq*sps.n  Phase=pi/2  SampleTime=Ts
  sin(wt) : Sin  Amplitude=sps.k  Frequency=2*pi*Freq*mate.n  SampleTime=Ts
  Mag : Outport  SampleTime=Ts  VectorParamsAs1DForOutWhenUnconnected=off
  Phase : Outport  Port=2  SampleTime=Ts  VectorParamsAs1DForOutWhenUnconnected=off
  wires:
  In/1 -> Product/1, Product1/1
  sin(wt)/1 -> Product/2
  Product/1 -> Discrete Mean value/1
  Discrete Mean value/1 -> Real-Imag to Complex/1  "Real"
  Discrete Mean value1/1 -> Real-Imag to Complex/2  "Imag"
  Complex to Magnitude-Angle/1 -> Mag/1
  Rad->Deg./1 -> Phase/1
  Real-Imag to Complex/1 -> Complex to Magnitude-Angle/1
  Complex to Magnitude-Angle/2 -> Rad->Deg./1
  cos(wt)/1 -> Product1/2
  Product1/1 -> Discrete Mean value1/1

== system simetranss/Misc/RMS ==
  In : Inport  SampleTime=Ts
  Constant : Constant  Value=TrueRMS
  Data Type Conversion : DataTypeConversion  OutDataTypeStr=boolean  SaturateOnIntegerOverflow=off  RndMeth=Floor
  Logical Operator : Logic  Operator=NOT  AllPortsSameDT=off  OutDataTypeStr=boolean
  "RMS " : Subsystem
  Switch : Switch  Criteria=u2 ~= 0  Threshold=0.5  SaturateOnIntegerOverflow=off  InputSameDT=off
  "TrueRMS " : Subsystem
  RMS : Outport  SampleTime=Ts  VectorParamsAs1DForOutWhenUnconnected=off
  wires:
  In/1 -> "TrueRMS "/1(In), "RMS "/1(In)
  Switch/1 -> RMS/1
  "TrueRMS "/1(RMS) -> Switch/1
  "RMS "/1(RMS) -> Switch/3
  Constant/1 -> Data Type Conversion/1
  Data Type Conversion/1 -> Logical Operator/1, "TrueRMS "/Enable, Switch/2
  Logical Operator/1 -> "RMS "/Enable

== system simetranss/Network decoupling/DCbus Vrecv ==
  Vc-z : Inport
  Controlled Voltage Source1 : fl_lib/Electrical/Electrical Sources/Controlled Voltage Source
  Current Sensor : fl_lib/Electrical/Electrical Sensors/Current Sensor
  PS-Simulink Converter : nesl_utility/PS-Simulink Converter  PhysicalDomain=network_engine_domain  SubClassName=ps_output  LeftPortType=input  RightPortType=output  PseudoPeriodic=off  Frequencies=[]  VectorFormat=inherit  Unit=inherit  AffineConversion=off
  Simulink-PS Converter : nesl_utility/Simulink-PS Converter  PhysicalDomain=network_engine_domain  SubClassName=ps_input  LeftPortType=input  RightPortType=output  PseudoPeriodic=off  Frequencies=[]  NoiseDistribution=none  NoiseParameters=[]  Unit=1  AffineConversion=off  FilteringAndDerivatives=provide  SimscapeFilterOrder=1  InputFilterTimeConstant=0.001  UdotUserProvided=0
  Unit Delay5 : UnitDelay  SampleTime=Ts  HasFrameUpgradeWarning=on
  V+z : PMIOPort  Side=Right
  V-z : PMIOPort  Port=2  Side=Right
  Idc : Outport
  wires:
  Unit Delay5/1 -> Idc/1
  PS-Simulink Converter/1 -> Unit Delay5/1
  Vc-z/1 -> Simulink-PS Converter/1
  connections:
  Simulink-PS Converter/RConn1 -- Controlled Voltage Source1/RConn1
  Controlled Voltage Source1/LConn1 -- Current Sensor/LConn1
  PS-Simulink Converter/LConn1 -- Current Sensor/RConn1
  Current Sensor/RConn2 -- V+z/RConn1
  Controlled Voltage Source1/RConn2 -- V-z/RConn1

== system simetranss/Network decoupling/DCbus Vsend ==
  Iin : Inport
  Controlled Current Source1 : fl_lib/Electrical/Electrical Sources/Controlled Current Source
  PS-Simulink Converter : nesl_utility/PS-Simulink Converter  PhysicalDomain=network_engine_domain  SubClassName=ps_output  LeftPortType=input  RightPortType=output  PseudoPeriodic=off  Frequencies=[]  VectorFormat=1-D array  Unit=V  AffineConversion=off
  Simulink-PS Converter : nesl_utility/Simulink-PS Converter  PhysicalDomain=network_engine_domain  SubClassName=ps_input  LeftPortType=input  RightPortType=output  PseudoPeriodic=off  Frequencies=[]  NoiseDistribution=none  NoiseParameters=[]  Unit=1  AffineConversion=off  FilteringAndDerivatives=provide  SimscapeFilterOrder=1  InputFilterTimeConstant=0.001  UdotUserProvided=0
  Unit Delay1 : UnitDelay  SampleTime=Ts  HasFrameUpgradeWarning=on
  Voltage Sensor : fl_lib/Electrical/Electrical Sensors/Voltage Sensor
  + : PMIOPort  Side=Left
  - : PMIOPort  Port=2  Side=Left
  Vc : Outport
  wires:
  PS-Simulink Converter/1 -> Unit Delay1/1
  Unit Delay1/1 -> Vc/1
  Iin/1 -> Simulink-PS Converter/1
  connections:
  -/RConn1 -- Voltage Sensor/RConn2 -- Controlled Current Source1/LConn1
  Voltage Sensor/RConn1 -- PS-Simulink Converter/LConn1
  +/RConn1 -- Voltage Sensor/LConn1 -- Controlled Current Source1/RConn2
  Simulink-PS Converter/RConn1 -- Controlled Current Source1/RConn1

== system simetranss/Network decoupling/MATE 3-phase Compensated Half-Stubline ==
  recv : Inport
  Compensate : Subsystem  mask(Artemis 3-phase Coupled Stubline Compensation Block){freq=FF, Rdiff=R_diff, Ldiff=L_diff, Cdiff=C_diff, Lcomp=L_comp, Rdamp=R_damp, Cdamp=C_damp}
      mask prompts: freq "Frequency"; Rdiff "Rdiff Resistance (ohms)"; Ldiff "Ldiff Inductance (H)"; Cdiff "Cdiff Capacitance (F)"; Lcomp "Compensating inductance"; Rdamp "Damping branch resistance"; Cdamp "Damping branch capacitance"
      mask help:
      | This block is used to compensate the spurious capacitive reactive power of the ARTEMiS 3-phase Coupled Stubline.
      |
      | All its parameters are computed and transfered from companion ARTEMiS 3-phase Coupled Stubline block.
      mask init:
      | currentBlock=gcb;
      | 
      | % Rdiffnum=reshape(sscanf(Rdiff,'%f'), [3,3]); % carefull about row vs.column wize
      | % Ldiffnum=reshape(sscanf(Ldiff,'%f'), [3,3]);
      | % Cdiffnum=reshape(sscanf(Cdiff,'%f'), [3,3]);
      | 
      | FF = freq;
      | RR = Rdiff;
      | LL = Ldiff;
      | CC = Cdiff;
      | L_comp=Lcomp;
      | R_damp=Rdamp;
      | C_damp=Cdamp;
      | 
      | 
      | 
      | % Fr=eval(get_param(gcb,'freq'));
      | % Cap=eval(get_param(gcb,'DPL_cap'));
      | % L_comp=1/((2*pi*Fr)^2*Cap);     % calculate compensating inductance
      | % R_damp=1e8;                     % set damping resistance to high value
      | % C_coupling=0;                   % set coupling capacitor to low value
      | % 
      | % Req=get_param(gcb,'damping_Req');
      | % 
      | % solvedString=['L=',num2str(L_comp),',  R=',num2str(R_damp),',  C=',num2str(C_coupling)];
      | %     
      | % set_param(gcb,'solvedValues',solvedString)
      | % 
      | % if strcmp(Req,'on')
      | %     Fr0=eval(get_param(gcb,'undamped_Freq'));
      | %     Fr=eval(get_param(gcb,'freq'));
      | %     w0=2*pi*Fr0;
      | %     w=2*pi*Fr;
      | %     w_peak=2*pi*100;         % Peak of impedance function magnitude selected at 
      | %                             % a frequency of 80 -100 Hz. See paper, section C.
      | %     
      | % %=========================================================================================
      | % %     Symbolic Solution of equations is commented out - use numeric solver fsolve() instead                            
      | %                            
      | % %     syms RR LL CC
      | % % 
      | % %     Cap=eval(get_param(gcb,'DPL_cap'));
      | % %     L_comp=1/((2*pi*Fr)^2*Cap);  
      | % % 
      | % %     eqns = [LL*sqrt(1+(w*RR*CC)^2)/sqrt((1-w^2*LL*CC)^2+(w*RR*CC)^2)==L_comp,...
      | % %             1/(LL*CC)==w_peak^2,...
      | % %             (RR*w0*CC)^4==(1+CC/Cap)^3];
      | % %     S = vpasolve(eqns,[LL CC RR],[L_comp Cap 100]); % Solve equation numerically with
      | % %                                                     % starting values L_comp,
      | % %                                                     % Cap, 100 (for resistor)
      | % %     
      | % %     R_damp=real(eval(S.RR));           % Solved value for damping resistor
      | % %     L_comp=real(eval(S.LL));           % solved value for inductance
      | % %     C_coupling=real(eval(S.CC));       % solved value for coupling capacitor
      | % %     zeta=0.5*(sqrt(1+CC/Cap)-1);       % damping ratio.
      | % %     
      | % %     solvedString=['L=',num2str(L_comp),',  R=',num2str(R_damp),',  C=',num2str(C_coupling)];
      | % %==============================================================================================
      | %   
      | % 	fun = @(x)[ x(1)*sqrt(1+(w*x(3)*x(2))^2)/sqrt((1-w^2*x(1)*x(2))^2+(w*x(3)*x(2))^2)-L_comp;
      | %                 1/(x(1)*x(2))-w_peak^2;
      | %                 (x(3)*w0*x(2))^4-(1+x(2)/Cap)^(3)];
      | % 
      | % 	x0 = [L_comp,Cap,100];              %starting values
      | % 	options = optimset( 'TolX',1e-6,'TolFun',1e-6,'Display','iter','MaxFunEvals',10000,'MaxIter',1000);
      | %       
      | % 	xSol = fsolve(fun,x0,options);      
      | % 
      | %     
      | %     L_comp=xSol(1);
      | % 	C_coupling=xSol(2);
      | % 	R_damp=xSol(3);
      | % %     a=(1+C_coupling/Cap);
      | % %     zeta=(sqrt(a)-1)/2;    
      | % 
      | % 
      | %      solvedString=['L=',num2str(L_comp),',  R=',num2str(R_damp),',  C=',num2str(C_coupling)];
      | %     
      | %      set_param(gcb,'solvedValues',solvedString)
      | % end
      mask Help: eval('open ARTEMiS_CompensatedStubline.pdf;');
      mask DialogControl Container2 Prompt: Solved Parameters
      mask Display: disp('StubComp')
  Pass : Subsystem  Commented=on  mask(Artemis 3-phase Coupled Stubline Compensation Block){freq=FF, Rdiff=R_diff, Ldiff=L_diff, Cdiff=C_diff, Lcomp=L_comp, Rdamp=R_damp, Cdamp=C_damp}
      mask prompts: freq "Frequency"; Rdiff "Rdiff Resistance (ohms)"; Ldiff "Ldiff Inductance (H)"; Cdiff "Cdiff Capacitance (F)"; Lcomp "Compensating inductance"; Rdamp "Damping branch resistance"; Cdamp "Damping branch capacitance"
      mask help:
      | This block is used to compensate the spurious capacitive reactive power of the ARTEMiS 3-phase Coupled Stubline.
      |
      | All its parameters are computed and transfered from companion ARTEMiS 3-phase Coupled Stubline block.
      mask init: same as simetranss/Network decoupling/MATE 3-phase Compensated Half-Stubline/Compensate
      mask Help: eval('open ARTEMiS_CompensatedStubline.pdf;');
      mask DialogControl Container2 Prompt: Solved Parameters
      mask Display: disp('StubComp')
  stubline : Subsystem
  abc : PMIOPort  Side=Right
  send : Outport
  wires:
  recv/1 -> stubline/1(hi)
  stubline/1(ho) -> send/1
  connections:
  abc/RConn1 -- Pass/LConn1 -- Compensate/LConn1
  Compensate/RConn1 -- Pass/RConn1 -- stubline/LConn1

== system simetranss/Network decoupling/RTScapeHalfStub ==
  note: SL1
  note: demistub
  hin : Inport
  Gain1 : Gain  Gain=h  SaturateOnIntegerOverflow=on  OutDataTypeStr=Inherit: Same as input  ParamDataTypeStr=Inherit: Same as input
  Gain2 : Gain  Gain=Z  SaturateOnIntegerOverflow=on  OutDataTypeStr=Inherit: Same as input  ParamDataTypeStr=Inherit: Same as input
  Gain3 : Gain  Gain=(1+h)./(Zm+Rt4)  SaturateOnIntegerOverflow=on  OutDataTypeStr=Inherit: Same as input  ParamDataTypeStr=Inherit: Same as input
  Gain4 : Gain  Gain=(1+h)/2  SaturateOnIntegerOverflow=on  OutDataTypeStr=Inherit: Same as input  ParamDataTypeStr=Inherit: Same as input
  Gain6 : Gain  Gain=(1-h)/2  SaturateOnIntegerOverflow=on  OutDataTypeStr=Inherit: Same as input  ParamDataTypeStr=Inherit: Same as input
  Signal Specification : SignalSpecification  Dimensions=1
  Simscape : Subsystem
      mask Display: disp('V')
  Sum1 : Sum  Inputs=+-  InputSameDT=on  SaturateOnIntegerOverflow=on  OutDataTypeStr=Inherit: Same as first input
  Sum3 : Sum  InputSameDT=on  SaturateOnIntegerOverflow=on  OutDataTypeStr=Inherit: Same as first input
  Unit Delay : UnitDelay  SampleTime=Ts  HasFrameUpgradeWarning=on
  Unit Delay1 : UnitDelay  SampleTime=Ts  HasFrameUpgradeWarning=on
  Voltage Source : Subsystem
  Z : ee_lib/Passive/Resistor  R=Z Ohm  enable_R_tol=ee.enum.toleranceApplication.none  R_tol=5  tol_distribution=ee.enum.toleranceDistribution.uniform  nSigma=4  enable_operating_limits=ee.enum.enable.no  operating_limit_action=ee.enum.passive.reportOpLim.warn  power_rating=1 W  max_working_voltage=100 V  noise_mode=ee.enum.sources.noise.Disabled  Tdevice=25 degC  sample_time=1e-3 s  repeatability=ee.enum.ic.repeatability.notRepeatable  user_seed=0  auto_seed=415452298  fault_action=simscape.enum.assert.action.none  t_fault=1 s  power_derating_T1=70 degC  power_derating_T2=155 degC  operating_temperature_range_vec=[-50, 150] degC  alpha=3.93e-3 1/K  Tmeas=25 degC  thermal_mass=100 J/K  temperature_specify=off  temperature_priority=High  temperature=298.15 K  temperature_nominal_specify=off  temperature_nominal_value=1  temperature_nominal_unit=K
  + : PMIOPort  Side=Left
  - : PMIOPort  Port=2  Side=Left
  hou : Outport  VectorParamsAs1DForOutWhenUnconnected=off
  wires:
  Unit Delay/1 -> hou/1
  Gain1/1 -> Sum1/2
  Gain3/1 -> Sum1/1
  [vt] -> Gain3/1
  Simscape/1(v) -> [vt]
  Signal Specification/1 -> [vin]
  [vin] -> Voltage Source/1(V)
  Sum1/1 -> Gain4/1, Gain6/1
  Gain6/1 -> Unit Delay1/1
  Gain4/1 -> Unit Delay/1
  Sum3/1 -> Gain1/1, Gain2/1
  Gain2/1 -> Signal Specification/1
  hin/1 -> Sum3/2
  Unit Delay1/1 -> Sum3/1
  connections:
  Voltage Source/RConn2 -- Simscape/LConn2 -- -/RConn1
  Simscape/LConn1 -- Z/RConn1 -- +/RConn1
  Z/LConn1 -- Voltage Source/RConn1
